simulink library "ddm"  (Simulink 8.2)
settings: Solver=ode45  SolverMode=SingleTasking  StartTime=0.0  StopTime=10.0  RelTol=1e-3
libraries: simulink x3
settings Model: Creator=R00T  LastModifiedBy=14014

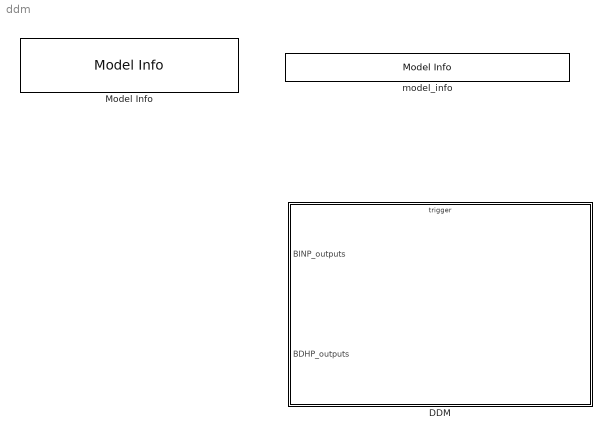
== system ddm ==
  DDM : Subsystem
      settings: RTWSystemCode=Nonreusable function  RTWFcnNameOpts=Use subsystem name  RTWFileNameOpts=Use subsystem name
  Model Info : simulink/Model-Wide Utilities/Model Info  InitialBlockCM=None  BlockCM=None  Frame=on  DisplayStringWithTags=|  HorizontalTextAlignment=Left  LeftAlignmentValue=0.02  SourceBlockDiagram=ddm  TagMaxNumber=20
      | Model Version        : %<ModelVersion>
      | Creator                   : %<Creator>
      | Last Modified by    : %<LastModifiedBy>
  model_info : simulink/Model-Wide Utilities/Model Info  InitialBlockCM=None  BlockCM=None  Frame=on  DisplayStringWithTags=$Id: hcu_lib.mdl 1464 2016-08-01 05:27:43Z chimotsai $  HorizontalTextAlignment=Center  LeftAlignmentValue=0.5  SourceBlockDiagram=ddm  TagMaxNumber=20

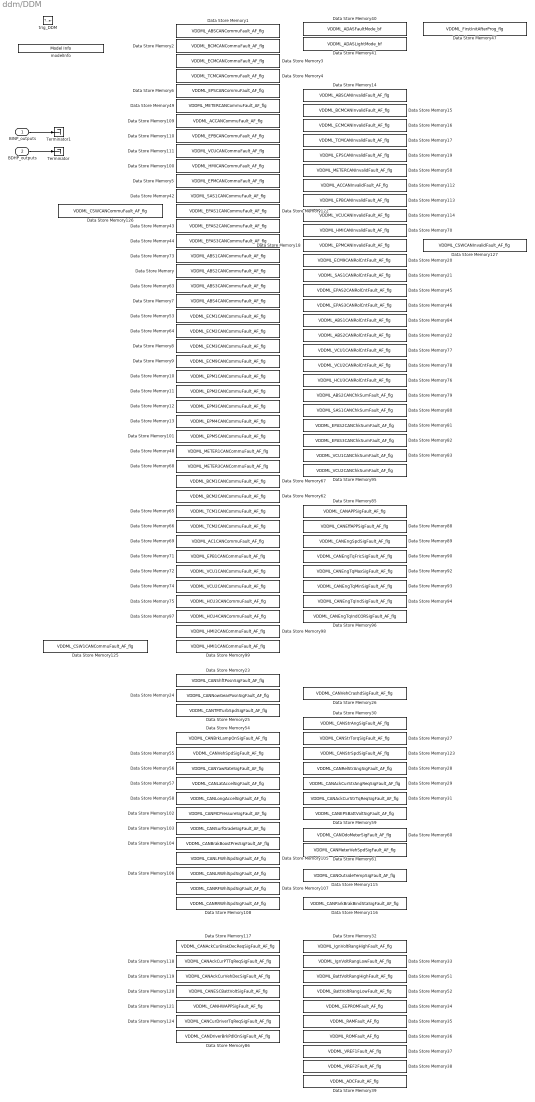
== system ddm/DDM ==
  BINP_outputs : Inport  OutDataTypeStr=Bus: BINP_outputs
  BDHP_outputs : Inport  Port=2
  trig_DDM : TriggerPort  TriggerType=function-call
  Data Store Memory : DataStoreMemory  DataStoreName=VDDML_ABS2CANCommuFault_AF_flg  WriteAfterWriteMsg=warning
  Data Store Memory1 : DataStoreMemory  DataStoreName=VDDML_ABSCANCommuFault_AF_flg  WriteAfterWriteMsg=warning
  Data Store Memory10 : DataStoreMemory  DataStoreName=VDDML_EPM1CANCommuFault_AF_flg  WriteAfterWriteMsg=warning
  Data Store Memory100 : DataStoreMemory  DataStoreName=VDDML_HMICANCommuFault_AF_flg  WriteAfterWriteMsg=warning
  Data Store Memory101 : DataStoreMemory  DataStoreName=VDDML_EPM5CANCommuFault_AF_flg  WriteAfterWriteMsg=warning
  Data Store Memory102 : DataStoreMemory  DataStoreName=VDDML_CANMCPressureSigFault_AF_flg  WriteAfterWriteMsg=warning
  Data Store Memory103 : DataStoreMemory  DataStoreName=VDDML_CANSurfGradeSigFault_AF_flg  WriteAfterWriteMsg=warning
  Data Store Memory104 : DataStoreMemory  DataStoreName=VDDML_CANBrakBoostPresSigFault_AF_flg  WriteAfterWriteMsg=warning
  Data Store Memory105 : DataStoreMemory  DataStoreName=VDDML_CANLFWhlSpdSigFault_AF_flg  WriteAfterWriteMsg=warning
  Data Store Memory106 : DataStoreMemory  DataStoreName=VDDML_CANLRWhlSpdSigFault_AF_flg  WriteAfterWriteMsg=warning
  Data Store Memory107 : DataStoreMemory  DataStoreName=VDDML_CANRFWhlSpdSigFault_AF_flg  WriteAfterWriteMsg=warning
  Data Store Memory108 : DataStoreMemory  DataStoreName=VDDML_CANRRWhlSpdSigFault_AF_flg  WriteAfterWriteMsg=warning
  Data Store Memory109 : DataStoreMemory  DataStoreName=VDDML_ACCANCommuFault_AF_flg  WriteAfterWriteMsg=warning
  Data Store Memory11 : DataStoreMemory  DataStoreName=VDDML_EPM2CANCommuFault_AF_flg  WriteAfterWriteMsg=warning
  Data Store Memory110 : DataStoreMemory  DataStoreName=VDDML_EPBCANCommuFault_AF_flg  WriteAfterWriteMsg=warning
  Data Store Memory111 : DataStoreMemory  DataStoreName=VDDML_VCUCANCommuFault_AF_flg  WriteAfterWriteMsg=warning
  Data Store Memory112 : DataStoreMemory  DataStoreName=VDDML_ACCANInvalidFault_AF_flg  WriteAfterWriteMsg=warning
  Data Store Memory113 : DataStoreMemory  DataStoreName=VDDML_EPBCANInvalidFault_AF_flg  WriteAfterWriteMsg=warning
  Data Store Memory114 : DataStoreMemory  DataStoreName=VDDML_VCUCANInvalidFault_AF_flg  WriteAfterWriteMsg=warning
  Data Store Memory115 : DataStoreMemory  DataStoreName=VDDML_CANOutsideTempSigFault_AF_flg  WriteAfterWriteMsg=warning
  Data Store Memory116 : DataStoreMemory  DataStoreName=VDDML_CANParkBrakBindStaSigFault_AF_flg  WriteAfterWriteMsg=warning
  Data Store Memory117 : DataStoreMemory  DataStoreName=VDDML_CANAckCurBrakDecReqSigFault_AF_flg  WriteAfterWriteMsg=warning
  Data Store Memory118 : DataStoreMemory  DataStoreName=VDDML_CANAckCurPTTqReqSigFault_AF_flg  WriteAfterWriteMsg=warning
  Data Store Memory119 : DataStoreMemory  DataStoreName=VDDML_CANAckCurVehDecSigFault_AF_flg  WriteAfterWriteMsg=warning
  Data Store Memory12 : DataStoreMemory  DataStoreName=VDDML_EPM3CANCommuFault_AF_flg  WriteAfterWriteMsg=warning
  Data Store Memory120 : DataStoreMemory  DataStoreName=VDDML_CANESCBattVoltSigFault_AF_flg  WriteAfterWriteMsg=warning
  Data Store Memory121 : DataStoreMemory  DataStoreName=VDDML_CANHWAPPSigFault_AF_flg  WriteAfterWriteMsg=warning
  Data Store Memory122 : DataStoreMemory  DataStoreName=VDDML_EPAS1CANCommuFault_AF_flg  WriteAfterWriteMsg=warning
  Data Store Memory123 : DataStoreMemory  DataStoreName=VDDML_CANStrSpdSigFault_AF_flg  WriteAfterWriteMsg=warning
  Data Store Memory124 : DataStoreMemory  DataStoreName=VDDML_CANCurDriverTqReqSigFault_AF_flg  WriteAfterWriteMsg=warning
  Data Store Memory125 : DataStoreMemory  DataStoreName=VDDML_CSW1CANCommuFault_AF_flg  WriteAfterWriteMsg=warning
  Data Store Memory126 : DataStoreMemory  DataStoreName=VDDML_CSWCANCommuFault_AF_flg  WriteAfterWriteMsg=warning
  Data Store Memory127 : DataStoreMemory  DataStoreName=VDDML_CSWCANInvalidFault_AF_flg  WriteAfterWriteMsg=warning
  Data Store Memory13 : DataStoreMemory  DataStoreName=VDDML_EPM4CANCommuFault_AF_flg  WriteAfterWriteMsg=warning
  Data Store Memory14 : DataStoreMemory  DataStoreName=VDDML_ABSCANInvalidFault_AF_flg  WriteAfterWriteMsg=warning
  Data Store Memory15 : DataStoreMemory  DataStoreName=VDDML_BCMCANInvalidFault_AF_flg  WriteAfterWriteMsg=warning
  Data Store Memory16 : DataStoreMemory  DataStoreName=VDDML_ECMCANInvalidFault_AF_flg  WriteAfterWriteMsg=warning
  Data Store Memory17 : DataStoreMemory  DataStoreName=VDDML_TCMCANInvalidFault_AF_flg  WriteAfterWriteMsg=warning
  Data Store Memory18 : DataStoreMemory  DataStoreName=VDDML_EPMCANInvalidFault_AF_flg  WriteAfterWriteMsg=warning
  Data Store Memory19 : DataStoreMemory  DataStoreName=VDDML_EPSCANInvalidFault_AF_flg  WriteAfterWriteMsg=warning
  Data Store Memory2 : DataStoreMemory  DataStoreName=VDDML_BCMCANCommuFault_AF_flg  WriteAfterWriteMsg=warning
  Data Store Memory20 : DataStoreMemory  DataStoreName=VDDML_ECM9CANRolCntFault_AF_flg  WriteAfterWriteMsg=warning
  Data Store Memory21 : DataStoreMemory  DataStoreName=VDDML_SAS1CANRolCntFault_AF_flg  WriteAfterWriteMsg=warning
  Data Store Memory22 : DataStoreMemory  DataStoreName=VDDML_ABS2CANRolCntFault_AF_flg  WriteAfterWriteMsg=warning
  Data Store Memory23 : DataStoreMemory  DataStoreName=VDDML_CANShftPosnSigFault_AF_flg  WriteAfterWriteMsg=warning
  Data Store Memory24 : DataStoreMemory  DataStoreName=VDDML_CANNowGearPosnSigFault_AF_flg  WriteAfterWriteMsg=warning
  Data Store Memory25 : DataStoreMemory  DataStoreName=VDDML_CANTMTurbSpdSigFault_AF_flg  WriteAfterWriteMsg=warning
  Data Store Memory26 : DataStoreMemory  DataStoreName=VDDML_CANVehCrashdSigFault_AF_flg  WriteAfterWriteMsg=warning
  Data Store Memory27 : DataStoreMemory  DataStoreName=VDDML_CANStrTorqSigFault_AF_flg  WriteAfterWriteMsg=warning
  Data Store Memory28 : DataStoreMemory  DataStoreName=VDDML_CANRelStrAngSigFault_AF_flg  WriteAfterWriteMsg=warning
  Data Store Memory29 : DataStoreMemory  DataStoreName=VDDML_CANAckCurStrAngReqSigFault_AF_flg  WriteAfterWriteMsg=warning
  Data Store Memory3 : DataStoreMemory  DataStoreName=VDDML_ECMCANCommuFault_AF_flg  WriteAfterWriteMsg=warning
  Data Store Memory30 : DataStoreMemory  DataStoreName=VDDML_CANStrAngSigFault_AF_flg  WriteAfterWriteMsg=warning
  Data Store Memory31 : DataStoreMemory  DataStoreName=VDDML_CANAckCurStrTqReqSigFault_AF_flg  WriteAfterWriteMsg=warning
  Data Store Memory32 : DataStoreMemory  DataStoreName=VDDML_IgnVoltRangHighFault_AF_flg  WriteAfterWriteMsg=warning
  Data Store Memory33 : DataStoreMemory  DataStoreName=VDDML_IgnVoltRangLowFault_AF_flg  WriteAfterWriteMsg=warning
  Data Store Memory34 : DataStoreMemory  DataStoreName=VDDML_EEPROMFault_AF_flg  WriteAfterWriteMsg=warning
  Data Store Memory35 : DataStoreMemory  DataStoreName=VDDML_RAMFault_AF_flg  WriteAfterWriteMsg=warning
  Data Store Memory36 : DataStoreMemory  DataStoreName=VDDML_ROMFault_AF_flg  WriteAfterWriteMsg=warning
  Data Store Memory37 : DataStoreMemory  DataStoreName=VDDML_VREF1Fault_AF_flg  WriteAfterWriteMsg=warning
  Data Store Memory38 : DataStoreMemory  DataStoreName=VDDML_VREF2Fault_AF_flg  WriteAfterWriteMsg=warning
  Data Store Memory39 : DataStoreMemory  DataStoreName=VDDML_ADCFault_AF_flg  WriteAfterWriteMsg=warning
  Data Store Memory4 : DataStoreMemory  DataStoreName=VDDML_TCMCANCommuFault_AF_flg  WriteAfterWriteMsg=warning
  Data Store Memory40 : DataStoreMemory  DataStoreName=VDDML_ADASFaultMode_bf  WriteAfterWriteMsg=warning
  Data Store Memory41 : DataStoreMemory  DataStoreName=VDDML_ADASLightMode_bf  WriteAfterWriteMsg=warning
  Data Store Memory42 : DataStoreMemory  DataStoreName=VDDML_SAS1CANCommuFault_AF_flg  WriteAfterWriteMsg=warning
  Data Store Memory43 : DataStoreMemory  DataStoreName=VDDML_EPAS2CANCommuFault_AF_flg  WriteAfterWriteMsg=warning
  Data Store Memory44 : DataStoreMemory  DataStoreName=VDDML_EPAS3CANCommuFault_AF_flg  WriteAfterWriteMsg=warning
  Data Store Memory45 : DataStoreMemory  DataStoreName=VDDML_EPAS2CANRolCntFault_AF_flg  WriteAfterWriteMsg=warning
  Data Store Memory46 : DataStoreMemory  DataStoreName=VDDML_EPAS3CANRolCntFault_AF_flg  WriteAfterWriteMsg=warning
  Data Store Memory47 : DataStoreMemory  DataStoreName=VDDML_FirstInitAfterProg_flg  WriteAfterWriteMsg=warning
  Data Store Memory48 : DataStoreMemory  DataStoreName=VDDML_METER1CANCommuFault_AF_flg  WriteAfterWriteMsg=warning
  Data Store Memory49 : DataStoreMemory  DataStoreName=VDDML_METERCANCommuFault_AF_flg  WriteAfterWriteMsg=warning
  Data Store Memory5 : DataStoreMemory  DataStoreName=VDDML_EPMCANCommuFault_AF_flg  WriteAfterWriteMsg=warning
  Data Store Memory50 : DataStoreMemory  DataStoreName=VDDML_METERCANInvalidFault_AF_flg  WriteAfterWriteMsg=warning
  Data Store Memory51 : DataStoreMemory  DataStoreName=VDDML_BattVoltRangHighFault_AF_flg  WriteAfterWriteMsg=warning
  Data Store Memory52 : DataStoreMemory  DataStoreName=VDDML_BattVoltRangLowFault_AF_flg  WriteAfterWriteMsg=warning
  Data Store Memory53 : DataStoreMemory  DataStoreName=VDDML_ECM1CANCommuFault_AF_flg  WriteAfterWriteMsg=warning
  Data Store Memory54 : DataStoreMemory  DataStoreName=VDDML_CANBrkLampOnSigFault_AF_flg  WriteAfterWriteMsg=warning
  Data Store Memory55 : DataStoreMemory  DataStoreName=VDDML_CANVehSpdSigFault_AF_flg  WriteAfterWriteMsg=warning
  Data Store Memory56 : DataStoreMemory  DataStoreName=VDDML_CANYawRateSigFault_AF_flg  WriteAfterWriteMsg=warning
  Data Store Memory57 : DataStoreMemory  DataStoreName=VDDML_CANLatAccelSigFault_AF_flg  WriteAfterWriteMsg=warning
  Data Store Memory58 : DataStoreMemory  DataStoreName=VDDML_CANLongAccelSigFault_AF_flg  WriteAfterWriteMsg=warning
  Data Store Memory59 : DataStoreMemory  DataStoreName=VDDML_CANEPSBattVoltSigFault_AF_flg  WriteAfterWriteMsg=warning
  Data Store Memory6 : DataStoreMemory  DataStoreName=VDDML_EPSCANCommuFault_AF_flg  WriteAfterWriteMsg=warning
  Data Store Memory60 : DataStoreMemory  DataStoreName=VDDML_CANOdoMeterSigFault_AF_flg  WriteAfterWriteMsg=warning
  Data Store Memory61 : DataStoreMemory  DataStoreName=VDDML_CANMeterVehSpdSigFault_AF_flg  WriteAfterWriteMsg=warning
  Data Store Memory62 : DataStoreMemory  DataStoreName=VDDML_BCM2CANCommuFault_AF_flg  WriteAfterWriteMsg=warning
  Data Store Memory63 : DataStoreMemory  DataStoreName=VDDML_ABS3CANCommuFault_AF_flg  WriteAfterWriteMsg=warning
  Data Store Memory64 : DataStoreMemory  DataStoreName=VDDML_ECM2CANCommuFault_AF_flg  WriteAfterWriteMsg=warning
  Data Store Memory65 : DataStoreMemory  DataStoreName=VDDML_TCM1CANCommuFault_AF_flg  WriteAfterWriteMsg=warning
  Data Store Memory66 : DataStoreMemory  DataStoreName=VDDML_TCM2CANCommuFault_AF_flg  WriteAfterWriteMsg=warning
  Data Store Memory67 : DataStoreMemory  DataStoreName=VDDML_BCM1CANCommuFault_AF_flg  WriteAfterWriteMsg=warning
  Data Store Memory68 : DataStoreMemory  DataStoreName=VDDML_METER3CANCommuFault_AF_flg  WriteAfterWriteMsg=warning
  Data Store Memory69 : DataStoreMemory  DataStoreName=VDDML_AC1CANCommuFault_AF_flg  WriteAfterWriteMsg=warning
  Data Store Memory7 : DataStoreMemory  DataStoreName=VDDML_ABS4CANCommuFault_AF_flg  WriteAfterWriteMsg=warning
  Data Store Memory70 : DataStoreMemory  DataStoreName=VDDML_HMICANInvalidFault_AF_flg  WriteAfterWriteMsg=warning
  Data Store Memory71 : DataStoreMemory  DataStoreName=VDDML_EPB1CANCommuFault_AF_flg  WriteAfterWriteMsg=warning
  Data Store Memory72 : DataStoreMemory  DataStoreName=VDDML_VCU1CANCommuFault_AF_flg  WriteAfterWriteMsg=warning
  Data Store Memory73 : DataStoreMemory  DataStoreName=VDDML_ABS1CANCommuFault_AF_flg  WriteAfterWriteMsg=warning
  Data Store Memory74 : DataStoreMemory  DataStoreName=VDDML_VCU2CANCommuFault_AF_flg  WriteAfterWriteMsg=warning
  Data Store Memory75 : DataStoreMemory  DataStoreName=VDDML_HCU3CANCommuFault_AF_flg  WriteAfterWriteMsg=warning
  Data Store Memory76 : DataStoreMemory  DataStoreName=VDDML_HCU3CANRolCntFault_AF_flg  WriteAfterWriteMsg=warning
  Data Store Memory77 : DataStoreMemory  DataStoreName=VDDML_VCU1CANRolCntFault_AF_flg  WriteAfterWriteMsg=warning
  Data Store Memory78 : DataStoreMemory  DataStoreName=VDDML_VCU2CANRolCntFault_AF_flg  WriteAfterWriteMsg=warning
  Data Store Memory79 : DataStoreMemory  DataStoreName=VDDML_ABS2CANChkSumFault_AF_flg  WriteAfterWriteMsg=warning
  Data Store Memory8 : DataStoreMemory  DataStoreName=VDDML_ECM3CANCommuFault_AF_flg  WriteAfterWriteMsg=warning
  Data Store Memory80 : DataStoreMemory  DataStoreName=VDDML_SAS1CANChkSumFault_AF_flg  WriteAfterWriteMsg=warning
  Data Store Memory81 : DataStoreMemory  DataStoreName=VDDML_EPAS2CANChkSumFault_AF_flg  WriteAfterWriteMsg=warning
  Data Store Memory82 : DataStoreMemory  DataStoreName=VDDML_EPAS3CANChkSumFault_AF_flg  WriteAfterWriteMsg=warning
  Data Store Memory83 : DataStoreMemory  DataStoreName=VDDML_VCU1CANChkSumFault_AF_flg  WriteAfterWriteMsg=warning
  Data Store Memory84 : DataStoreMemory  DataStoreName=VDDML_ABS1CANRolCntFault_AF_flg  WriteAfterWriteMsg=warning
  Data Store Memory85 : DataStoreMemory  DataStoreName=VDDML_CANAPPSigFault_AF_flg  WriteAfterWriteMsg=warning
  Data Store Memory86 : DataStoreMemory  DataStoreName=VDDML_CANDriverBrkPdlOnSigFault_AF_flg  WriteAfterWriteMsg=warning
  Data Store Memory88 : DataStoreMemory  DataStoreName=VDDML_CANEffAPPSigFault_AF_flg  WriteAfterWriteMsg=warning
  Data Store Memory89 : DataStoreMemory  DataStoreName=VDDML_CANEngSpdSigFault_AF_flg  WriteAfterWriteMsg=warning
  Data Store Memory9 : DataStoreMemory  DataStoreName=VDDML_ECM9CANCommuFault_AF_flg  WriteAfterWriteMsg=warning
  Data Store Memory90 : DataStoreMemory  DataStoreName=VDDML_CANEngTqFricSigFault_AF_flg  WriteAfterWriteMsg=warning
  Data Store Memory92 : DataStoreMemory  DataStoreName=VDDML_CANEngTqMaxSigFault_AF_flg  WriteAfterWriteMsg=warning
  Data Store Memory93 : DataStoreMemory  DataStoreName=VDDML_CANEngTqMinSigFault_AF_flg  WriteAfterWriteMsg=warning
  Data Store Memory94 : DataStoreMemory  DataStoreName=VDDML_CANEngTqIndSigFault_AF_flg  WriteAfterWriteMsg=warning
  Data Store Memory95 : DataStoreMemory  DataStoreName=VDDML_VCU2CANChkSumFault_AF_flg  WriteAfterWriteMsg=warning
  Data Store Memory96 : DataStoreMemory  DataStoreName=VDDML_CANEngTqIndCORSigFault_AF_flg  WriteAfterWriteMsg=warning
  Data Store Memory97 : DataStoreMemory  DataStoreName=VDDML_HCU4CANCommuFault_AF_flg  WriteAfterWriteMsg=warning
  Data Store Memory98 : DataStoreMemory  DataStoreName=VDDML_HMI2CANCommuFault_AF_flg  WriteAfterWriteMsg=warning
  Data Store Memory99 : DataStoreMemory  DataStoreName=VDDML_HMI1CANCommuFault_AF_flg  WriteAfterWriteMsg=warning
  Terminator : Terminator
  Terminator1 : Terminator
  modelInfo : simulink/Model-Wide Utilities/Model Info  InitialBlockCM=None  BlockCM=None  Frame=on  DisplayStringWithTags=%<ModifiedDate>  HorizontalTextAlignment=Center  LeftAlignmentValue=0.5  SourceBlockDiagram=ddm  TagMaxNumber=20
  wires:
  BDHP_outputs/1 -> Terminator/1
  BINP_outputs/1 -> Terminator1/1
